simulink model "iddempr2"  (Simulink 4.00)
settings: Solver=ode45  StartTime=0.0  StopTime=500  RelTol=1e-3
settings Model: Creator=ljung  LimitDataPoints=off  IntegerOverflowMsg=none  ExtModeTrigMode=oneshot  ExtModeArmWhenConnect=off  ExtModeAutoUpdateStatusClock=off

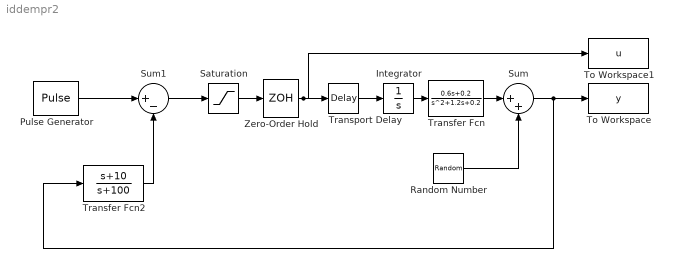
== system iddempr2 ==
  Integrator : Integrator  ExternalReset=none  InitialConditionSource=internal  InitialCondition=0  LimitOutput=off  UpperSaturationLimit=inf  LowerSaturationLimit=-inf  ShowSaturationPort=off  ShowStatePort=off  AbsoluteTolerance=auto
  Pulse Generator : DiscretePulseGenerator  PulseType=Sample-based  Amplitude=1  Period=200  PulseWidth=50  PhaseDelay=0  SampleTime=1
  Random Number : RandomNumber  Mean=0  Variance=0.1  Seed=0  SampleTime=1
  Saturation : Saturate  UpperLimit=0.5  LowerLimit=-0.5  LinearizeAsGain=on
  Sum : Sum  Inputs=|++  SaturateOnIntegerOverflow=on
  Sum1 : Sum  Inputs=|+-  SaturateOnIntegerOverflow=on
  To Workspace : ToWorkspace  VariableName=y  SampleTime=1  SaveFormat=Array
  To Workspace1 : ToWorkspace  VariableName=u  SampleTime=1  SaveFormat=Array
  Transfer Fcn : TransferFcn  Numerator=[0.6 0.2]  Denominator="[1 1.2  0.2]"  AbsoluteTolerance=auto  Realization=auto
  Transfer Fcn2 : TransferFcn  Numerator=[1 10]  Denominator=[1 100]  AbsoluteTolerance=auto  Realization=auto
  Transport Delay : TransportDelay  DelayTime=2.2  InitialInput=0  BufferSize=1024  PadeOrder=0
  Zero-Order Hold : ZeroOrderHold  SampleTime=1
  wires:
  Transfer Fcn/1 -> Sum/1
  Random Number/1 -> Sum/2
  Sum/1 -> To Workspace/1, Transfer Fcn2/1
  Zero-Order Hold/1 -> To Workspace1/1, Transport Delay/1
  Transport Delay/1 -> Integrator/1
  Integrator/1 -> Transfer Fcn/1
  Sum1/1 -> Saturation/1
  Saturation/1 -> Zero-Order Hold/1
  Transfer Fcn2/1 -> Sum1/2
  Pulse Generator/1 -> Sum1/1
